simulink model "pump_simulator"  (R2020b)
settings: Solver=ode23t  StartTime=0.0  StopTime=sim_time  FixedStep=6.0  MaxStep=6.0  RelTol=1e-3
values from neighbouring files (symbols this model uses):
  bolus_size = 10    [insulin_pump.m]
  bolus_time = 3600*3    (= 10800)    [insulin_pump.m]
  damper_d1 = 5.0e4    (= 50000)    [insulin_pump.m]
  damper_d2 = 5    [insulin_pump.m]
  iis_area = pi*iis_diameter^2    (= 3.14159265359)    [insulin_pump.m]
  iis_elevation = 0    [insulin_pump.m]
  m_pulse_period = 3600 / n_pulses_per_hour    (= 180)    [insulin_pump.m]
  m_rotor_inertia = 0.051    [insulin_pump.m]
  m_volt = m_volt_nom    (= 3)    [insulin_pump.m]
  occ_area = iis_area    (= 3.14159265359)    [insulin_pump.m]
  occ_sw = 1    [insulin_pump.m]
  occ_tau = 2000    [insulin_pump.m]
  occ_time = s_locs(occ_idx)    [detect_occlusion.m]    (also in insulin_pump.m = 7200)
  piston_area = pi*reservoir_radius^2    [insulin_pump.m]
  piston_displacement_per_unit = U_per_ml / (piston_area)    [insulin_pump.m]
  piston_length = reservoir_len    (= 2.5)    [insulin_pump.m]
  pump_stop_time = 3600*6    (= 21600)    [insulin_pump.m]
  s_per_U = 60/flow_ml_min / 100    (= 12)    [insulin_pump.m]
  sim_time = 3600 * 10    (= 36000)    [insulin_pump.m]
  u_per_basal_pulse = basal_rate / n_pulses_per_hour    (= 0.05)    [insulin_pump.m]
libraries: fl_lib x38, nesl_utility x28, sh_lib x11, ee_lib x4, sdl_lib x3, simulink x1
(part 1 of 2)
Description:
  | Simulation of the physical mechanisms of an insulin pump.
settings Model: Creator=Mads  LastModifiedBy=Mads
settings DebuggingCC: AlgebraicLoopMsg=none

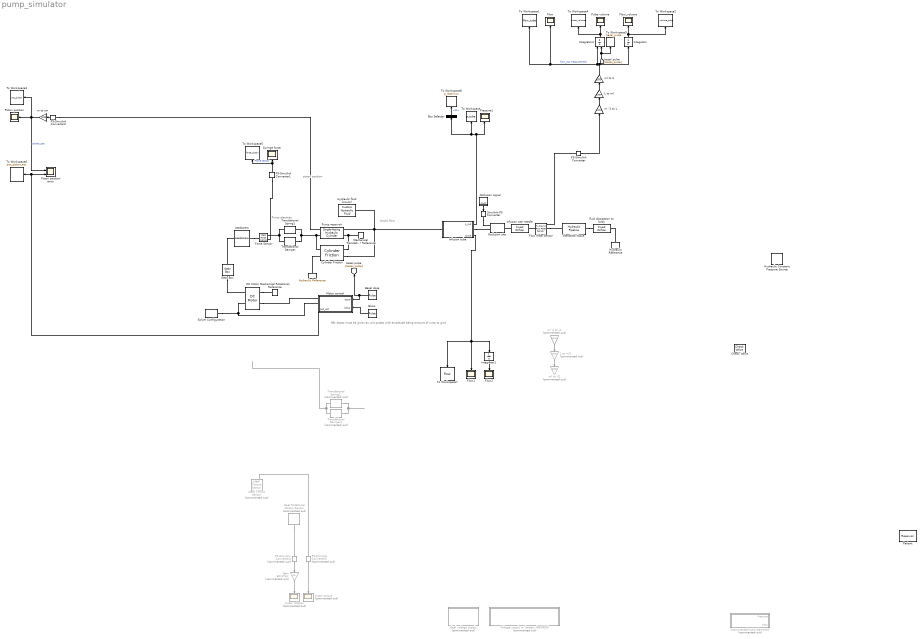
== system pump_simulator ==
  note: piston position
  note: NB: doses must be given as unit pulses with amplitude being amount of units to give
  note: Pump elasticity
  note: Insulin flow
  "  " : fl_lib/Hydraulic/Hydraulic Elements/Hydraulic Reference
  Basal dose : DiscretePulseGenerator  PulseType=Time based  Amplitude=u_per_basal_pulse  Period=m_pulse_period  PulseWidth=1e-11  PhaseDelay=10
  Bolus : DiscretePulseGenerator  PulseType=Time based  Amplitude=bolus_size  Period=sim_time  PulseWidth=1e-12  PhaseDelay=bolus_time
  Bus Selector : BusSelector  OutputSignals=p1
  Check Valve : sh_lib/Valves/Directional Valves/Check Valve  area_max=1e-4 m^2  pres_crack=0.3e5 Pa  pres_max=1.2e5 Pa  C_d=0.7  A_leak=1e-12 m^2  lam_spec=1  B_lam=0.999  Re_cr=12  dynamic=0  tau=0.1 s  area_init=1e-12 m^2
      settings: SourceProductBaseCode=SH  InternalSimscapePortConfiguration="{\"Bottom\":[],\"Left\":[{\"id\":\"A\",\"label\":\"A\",\"type\":\"foundation.hydraulic.hydraulic\"}],\"Right\":[{\"id\":\"B\",\"label\":\"B\",\"type\":\"foundation.hydraulic.hydraulic\"}],\"Top\":[]}"
  "Cylinder Friction " : sh_lib/Hydraulic Cylinders/Cylinder Friction  frc_preload=f_c N  fr_coef=f_cp N/Pa  frc_brkwy_coef=f_brk_c  visc_coef=f_v N/(m/s)  trans_coef=10000 s/m  vel_thr=v_limit cm/s  flow_rate_A_specify=off  flow_rate_A_priority=None  flow_rate_A=0 m^3/s  flow_rate_A_nominal_specify=off  flow_rate_A_nominal_unit=m^3/s  flow_rate_A_nominal_value=1  flow_rate_B_specify=off  flow_rate_B_priority=None  flow_rate_B=0 m^3/s  flow_rate_B_nominal_specify=off  flow_rate_B_nominal_unit=m^3/s  flow_rate_B_nominal_value=1  friction_force_specify=off  friction_force_priority=None  friction_force=0 N  friction_force_nominal_specify=off  friction_force_nominal_unit=N  friction_force_nominal_value=1  rel_velocity_specify=off  rel_velocity_priority=None  rel_velocity=0 m/s  rel_velocity_nominal_specify=off  rel_velocity_nominal_unit=m/s  rel_velocity_nominal_value=1
      settings: SourceProductBaseCode=SH  InternalSimscapePortConfiguration="{\"Bottom\":[],\"Left\":[{\"id\":\"A\",\"label\":\"A\",\"type\":\"foundation.hydraulic.hydraulic\"},{\"id\":\"C\",\"label\":\"C\",\"type\":\"foundation.mechanical.translational.translational\"}],\"Right\":[{\"id\":\"B\",\"label\":\"B\",\"type\":\"foundation.hydraulic.hydraulic\"},{\"id\":\"R\",\"label\":\"R\",\"type\":\"foundation.mechanical.translational.translational\"}],\"Top\":[]}"
  "DC Motor " : ee_lib/Electromechanical/Brushed Motors/DC Motor  field_option=ee.enum.field_option.pm  Rf=100 Ohm  Lf=1 H  Laf=0.15 H  If0=0 A  parameterization=ee.enum.dcparam_option.circuit_param  Ra=m_arm_res Ohm  La=m_arm_inductance uH  emf_or_torque=ee.enum.emf_or_torque.kv  Kv=m_back_emf V/rpm  Ki=6.876e-4 N*m/A  T_stall=0.24e-3 N*m  w_max=19100 rpm  w_rated=15000 rpm  P_rated=0.08 W  V_rated=1.5 V  J=m_rotor_inertia g*cm^2  lam_param=ee.enum.lam_param.damping  lam=0 N*m/(rad/s)  i_noload=0 A  V_i_noload=1.5 V  speed0=0 rpm  enable_fault_armature=ee.enum.faults.faultEnable.no  rev_faulted=1 / 3  G_faulted_armature=1e-5 S  fault_trigger_armature=ee.enum.faults.faultTrigger.temporal  t_fault_armature=1 s  max_permissible_current_armature=inf A  t_fail_on_current_armature=1 s  enable_fault_field=ee.enum.faults.faultEnable.no  G_faulted_field=1e-5 S  fault_trigger_field=ee.enum.faults.faultTrigger.temporal  t_fault_field=1 s  max_permissible_current_field=inf A  t_fail_on_current_field=1 s  fault_action=ee.enum.faults.faultAction.none  alpha=3.93e-3 1/K  Tmeas=25 degC  thermal_mass=100 J/K  initial_temperature=25 degC
  Flow : Scope
  Flow Rate Sensor : fl_lib/Hydraulic/Hydraulic Sensors/Hydraulic Flow Rate Sensor
  Flow1 : Scope
  Flow2 : Scope
  Flow_volume : Scope
  Force Sensor : fl_lib/Mechanical/Mechanical Sensors/Ideal Force Sensor
  Gain : Gain  Commented=on  Gain=60/(2*pi)
  "Gear Box " : fl_lib/Mechanical/Mechanisms/Gear Box  ratio=gear_ratio  t_in_specify=off  t_in_priority=None  t_in=0 N*m  t_in_nominal_specify=off  t_in_nominal_unit=N*m  t_in_nominal_value=1  t_out_specify=off  t_out_priority=None  t_out=0 N*m  t_out_nominal_specify=off  t_out_nominal_unit=N*m  t_out_nominal_value=1
  Hydraulic Constant Pressure Source : fl_lib/Hydraulic/Hydraulic Sources/Hydraulic Constant Pressure Source  commanded_pressure=patient_pressure Pa
      settings: SourceProductBaseCode=SS  InternalSimscapePortConfiguration="{\"Bottom\":[],\"Left\":[{\"id\":\"P\",\"label\":\"P\",\"type\":\"foundation.hydraulic.hydraulic\"}],\"Right\":[{\"id\":\"T\",\"label\":\"T\",\"type\":\"foundation.hydraulic.hydraulic\"}],\"Top\":[]}"
  "Hydraulic Reference " : fl_lib/Hydraulic/Hydraulic Elements/Hydraulic Reference
  Hydraulic fluid (insulin) : fl_lib/Hydraulic/Hydraulic Utilities/Custom Hydraulic Fluid  density=f_density kg/m^3  viscosity_kin=f_viscosity m^2/s  bulk=f_bmodulus GPa  alpha=0.005  range_error=2
      settings: SourceProductBaseCode=SS  InternalSimscapePortConfiguration="{\"Bottom\":[],\"Left\":[],\"Right\":[{\"id\":\"G\",\"label\":\"\",\"type\":\"foundation.hydraulic.hydraulic\"}],\"Top\":[]}"
  Ideal Rotational Motion Sensor : fl_lib/Mechanical/Mechanical Sensors/Ideal Rotational Motion Sensor  Commented=on  wrap_angle=simscape.enum.onoff.off  offset=0 rad
  Ideal Torque Sensor : fl_lib/Mechanical/Mechanical Sensors/Ideal Torque Sensor  Commented=on
  Ideal voltage supply : Subsystem  Commented=on
  Infusion site needle : sh_lib/Orifices/Fixed Orifice  area=cannula_area mm^2  C_d=0.7  lam_spec=1  B_lam=0.999  Re_cr=12  q_specify=off  q_priority=None  q=0.001 m^3/s  q_nominal_specify=off  q_nominal_unit=m^3/s  q_nominal_value=1  p_specify=on  p_priority=None  p=patient_pressure Pa  p_nominal_specify=off  p_nominal_unit=Pa  p_nominal_value=1
      settings: SourceProductBaseCode=SH  InternalSimscapePortConfiguration="{\"Bottom\":[],\"Left\":[{\"id\":\"A\",\"label\":\"A\",\"type\":\"foundation.hydraulic.hydraulic\"}],\"Right\":[{\"id\":\"B\",\"label\":\"B\",\"type\":\"foundation.hydraulic.hydraulic\"}],\"Top\":[]}"
  Infusion tube : Subsystem
      settings: PortSchema="{\"entries\":[{\"content\":{\"sides\":[{\"content\":{\"connectorIds\":[\"LConn1\"]},\"type\":\"ConnectorPlacement.EquallySpacedRectSide\",\"uuid\":\"e70f1e6d-11cd-47d8-af3d-56e3f4a89399\"},{\"content\":{\"connectorIds\":[\"Out1\",\"RConn1\",\"Out2\"],\"side\":\"RIGHT\"},\"type\":\"ConnectorPlacement.EquallySpacedRectSide\",\"uuid\":\"9455abbe-f67f-4bf6-bddd-a052e413b073\"},{\"content\":{\"connectorIds\":[],\"side\":\"TOP\"},\"type\":\"ConnectorPlacement.EquallySpacedRectSide\",\"uuid\":\"7aa9b125-01ea-4305-b1e3-58feaaf15538\"},{\"content\":{\"connectorIds\":[],\"side\":\"HIDDEN\"},\"type\":\"ConnectorPlacement.EquallySpacedRectSide\",\"uuid\":\"f40c7cd6-f259-44f6-9988-6f35709dc079\"}]},\"type\":\"ConnectorPlacement.EquallySpacedConnector\",\"uuid\":\"14f398f0-e936-4cfd-8d2f-f38c63dcd4d0\"}],\"packageUris\":[\"http://schema.mathworks.com/mf0/Connector/R2020b\"],\"version\":\"1.0\"}"
  Instrumented tube element3 : Subsystem  Commented=on
      settings: PortSchema="{\"entries\":[{\"content\":{\"sides\":[{\"content\":{\"connectorIds\":[\"LConn1\"]},\"type\":\"ConnectorPlacement.EquallySpacedRectSide\",\"uuid\":\"90113306-d748-46db-abc8-91bd69636f02\"},{\"content\":{\"connectorIds\":[\"Out1\",\"RConn1\",\"Out2\"],\"side\":\"RIGHT\"},\"type\":\"ConnectorPlacement.EquallySpacedRectSide\",\"uuid\":\"530dcab3-c363-40af-a674-d98a45a6a67f\"},{\"content\":{\"connectorIds\":[],\"side\":\"TOP\"},\"type\":\"ConnectorPlacement.EquallySpacedRectSide\",\"uuid\":\"49317322-7354-4795-83a8-239f759f7c98\"},{\"content\":{\"connectorIds\":[],\"side\":\"HIDDEN\"},\"type\":\"ConnectorPlacement.EquallySpacedRectSide\",\"uuid\":\"2a1d342c-23bd-4634-892a-7801d88aaf7b\"}]},\"type\":\"ConnectorPlacement.EquallySpacedConnector\",\"uuid\":\"7465f97d-dcd1-4a1e-863d-c659d9c7a8a5\"}],\"packageUris\":[\"http://schema.mathworks.com/mf0/Connector/R2020b\"],\"version\":\"1.0\"}"
  Integrator : Integrator
  Integrator1 : Integrator
  Integrator4 : Integrator  ExternalReset=rising
  Interstitial tissue : sh_lib/Pipelines/Hydraulic Pipeline  cs_type=1  d_in=pat_area m  area=1e-4 m^2  D_h=1.12e-2 m  s_factor=64  length=pat_len m  length_ad=pat_len m  roughness=15e-3 m  Re_lam=2000  Re_turb=4000  wall_type=2  pr_r_coef=pat_pressure_diameter m/Pa  time_const=pat_tau s  k_sh=1.4  initial_pressure=patient_pressure Pa
      settings: SourceProductBaseCode=SH  InternalSimscapePortConfiguration="{\"Bottom\":[],\"Left\":[{\"id\":\"A\",\"label\":\"A\",\"type\":\"foundation.hydraulic.hydraulic\"}],\"Right\":[{\"id\":\"B\",\"label\":\"B\",\"type\":\"foundation.hydraulic.hydraulic\"}],\"Top\":[]}"
  L to ml : Gain  Gain=1000
  L to ml1 : Gain  Commented=on  Gain=1000
  "Leadscrew " : sdl_lib/Gears/Rotational- Translational/Leadscrew  Lead=screw_lead cm  helix_type=sdl.enum.handedness.right  mu_visc=0 N*m/(rad/s)  friction_model=sdl.enum.gear_friction.constant  friction_parameterization=sdl.enum.frictionParameterization.geometry  lambda=15 deg  alpha=14.5 deg  fr_coeff=0.08  eff_sn=0.75  eff_ns=0.45  temperature_TLU=[280, 300, 320] K  efficiency_sn_TLU=[.75, .65, .6]  efficiency_ns_TLU=[.5, .45, .4]  pwr_thr=0.001 W  thermal_mass=50 J/K  temperature_specify=off  temperature_priority=High  temperature=300 K  temperature_nominal_specify=off  temperature_nominal_unit=K  temperature_nominal_value=1
      settings: SourceProductBaseCode=LD  InternalSimscapePortConfiguration="{\"Bottom\":[],\"Left\":[{\"id\":\"S\",\"label\":\"S\",\"type\":\"foundation.mechanical.rotational.rotational\"}],\"Right\":[{\"id\":\"N\",\"label\":\"N\",\"type\":\"foundation.mechanical.translational.translational\"}],\"Top\":[]}"
  Mechanical Rotational Reference : fl_lib/Mechanical/Rotational Elements/Mechanical Rotational Reference
  Mechanical Translational Reference : fl_lib/Mechanical/Translational Elements/Mechanical Translational Reference
  Motor control : Subsystem
      settings: PortSchema="{\"entries\":[{\"content\":{\"sides\":[{\"content\":{\"connectorIds\":[\"In1\",\"In2\"]},\"type\":\"ConnectorPlacement.EquallySpacedRectSide\",\"uuid\":\"d31ed946-0000-42cb-ba35-acda5a1e69b3\"},{\"content\":{\"connectorIds\":[\"RConn1\",\"RConn2\",\"Out1\"],\"side\":\"RIGHT\"},\"type\":\"ConnectorPlacement.EquallySpacedRectSide\",\"uuid\":\"d7d1f491-0bec-4320-8848-206ef8953605\"},{\"content\":{\"connectorIds\":[],\"side\":\"TOP\"},\"type\":\"ConnectorPlacement.EquallySpacedRectSide\",\"uuid\":\"d987aef5-87ba-45f9-8852-506aa6bf395c\"},{\"content\":{\"connectorIds\":[],\"side\":\"BOTTOM\"},\"type\":\"ConnectorPlacement.EquallySpacedRectSide\",\"uuid\":\"97925f89-ba97-42d0-b299-b4741c535cef\"},{\"content\":{\"connectorIds\":[],\"side\":\"HIDDEN\"},\"type\":\"ConnectorPlacement.EquallySpacedRectSide\",\"uuid\":\"d0973534-b90c-4eda-9531-680b99c38f66\"}]},\"type\":\"ConnectorPlacement.EquallySpacedConnector\",\"uuid\":\"4ca74101-9d3f-4e35-bde6-be4c600fefd9\"}],\"packageUris\":[\"http://schema.mathworks.com/mf0/Connector/R2020b\"],\"version\":\"1.0\"}"
  Occlusion signal : Subsystem
  Occlusion site : fl_lib/Hydraulic/Hydraulic Elements/Variable Area Hydraulic Orifice  C_d=0.7  min_area=1e-12 mm^2  lam_spec=1  B_lam=0.999  Re_cr=12  q_specify=off  q_priority=None  q=0.001 m^3/s  q_nominal_specify=off  q_nominal_unit=m^3/s  q_nominal_value=1  p_specify=off  p_priority=None  p=patient_pressure Pa  p_nominal_specify=off  p_nominal_unit=Pa  p_nominal_value=1
      settings: SourceProductBaseCode=SS  InternalSimscapePortConfiguration="{\"Bottom\":[],\"Left\":[{\"id\":\"AR\",\"label\":\"AR\",\"type\":\"input\"},{\"id\":\"A\",\"label\":\"A\",\"type\":\"foundation.hydraulic.hydraulic\"}],\"Right\":[{\"id\":\"B\",\"label\":\"B\",\"type\":\"foundation.hydraulic.hydraulic\"}],\"Top\":[]}"
  PS-Simulink Converter : nesl_utility/PS-Simulink Converter  PhysicalDomain=network_engine_domain  SubClassName=ps_output  LeftPortType=input  RightPortType=output  PseudoPeriodic=off  Frequencies=[]  Unit=inherit  AffineConversion=off
  PS-Simulink Converter1 : nesl_utility/PS-Simulink Converter  PhysicalDomain=network_engine_domain  SubClassName=ps_output  LeftPortType=input  RightPortType=output  PseudoPeriodic=off  Frequencies=[]  Unit=inherit  AffineConversion=off
  PS-Simulink Converter3 : nesl_utility/PS-Simulink Converter  PhysicalDomain=network_engine_domain  SubClassName=ps_output  LeftPortType=input  RightPortType=output  PseudoPeriodic=off  Frequencies=[]  Unit=inherit  AffineConversion=off
  PS-Simulink Converter4 : nesl_utility/PS-Simulink Converter  Commented=on  PhysicalDomain=network_engine_domain  SubClassName=ps_output  LeftPortType=input  RightPortType=output  PseudoPeriodic=off  Frequencies=[]  Unit=inherit  AffineConversion=off
  PS-Simulink Converter5 : nesl_utility/PS-Simulink Converter  Commented=on  PhysicalDomain=network_engine_domain  SubClassName=ps_output  LeftPortType=input  RightPortType=output  PseudoPeriodic=off  Frequencies=[]  Unit=inherit  AffineConversion=off
  Patient : sh_lib/Hydraulic Utilities/Reservoir  press=patient_pressure Pa  init_volume=5 l  ret_diam=cannula_area mm  loss_coeff=1
      settings: SourceProductBaseCode=SH  InternalSimscapePortConfiguration="{\"Bottom\":[],\"Left\":[{\"id\":\"V\",\"label\":\"V\",\"type\":\"output\"},{\"id\":\"P\",\"label\":\"P\",\"type\":\"foundation.hydraulic.hydraulic\"},{\"id\":\"R\",\"label\":\"R\",\"type\":\"foundation.hydraulic.hydraulic\"}],\"Right\":[],\"Top\":[]}"
  Piston position : Scope
  Piston position error : Scope  NumInputPorts=2
  Pressure1 : Scope
  Pulse volume : Scope
  Pump reservoir : sh_lib/Hydraulic Cylinders/Single-Acting Hydraulic Cylinder  area=piston_area cm^2  stroke=piston_length cm  init_pos=piston_length cm  dead_vol=piston_area*1e-12 cm^3  init_pressure=patient_pressure Pa  k_sh=1.4  stiff=1e6 N/m  D=150 N/(m/s)  hardstop_model=1  transition=4e-5 cm  or=2
      settings: SourceProductBaseCode=SH  InternalSimscapePortConfiguration="{\"Bottom\":[],\"Left\":[{\"id\":\"C\",\"label\":\"C\",\"type\":\"foundation.mechanical.translational.translational\"},{\"id\":\"A\",\"label\":\"A\",\"type\":\"foundation.hydraulic.hydraulic\"}],\"Right\":[{\"id\":\"R\",\"label\":\"R\",\"type\":\"foundation.mechanical.translational.translational\"},{\"id\":\"P\",\"label\":\"P\",\"type\":\"output\"}],\"Top\":[]}"
  Simulink-PS Converter : nesl_utility/Simulink-PS Converter  PhysicalDomain=network_engine_domain  SubClassName=ps_input  LeftPortType=input  RightPortType=output  PseudoPeriodic=off  Frequencies=[]  NoiseDistribution=none  NoiseParameters=[]  Unit=1  AffineConversion=off  FilteringAndDerivatives=provide  SimscapeFilterOrder=1  InputFilterTimeConstant=0.001  UdotUserProvided=0
  "Solver Configuration " : nesl_utility/Solver Configuration  PhysicalDomain=network_engine_domain  SubClassName=solver  LeftPortType=input  RightPortType=generic  Tones=[]  Harmonics=[]  SimulateNoise=off  Profile=off  UseLocalSampling=off  EnableSwitchedLinearOptims=on  FrequencyDomain=off  UseCCode=off  RelTol=0.001  AbsTol=1e-06  MinStep=1e-09  ToWorkspace=off  RevertToSquareIcSolve=off  NumHomotopyIterations=100  PhasorMode=off  PhasorModeNumHarmonics=1  DoDC=on  ResidualTolerance=1e-09  UseLocalSolver=off  LocalSolverChoice=NE_BACKWARD_EULER_ADVANCER  LocalSolverSampleTime=0.1  DoFixedCost=off  MaxNonlinIter=3  MaxModeIter=2  ComputeImpulses=off  ImpulseIterations=2  LinearAlgebra=auto  EquationFormulation=NE_TIME_EF  DelaysMemoryBudget=1024  AutomaticFiltering=on  FilteringTimeConstant=0.001  PartitionStorageMethod=AS_NEEDED  PartitionMemoryBudget=1024  PartitionMethod=ROBUST
  Syringe force : Scope
  To Workspace : ToWorkspace  VariableName=p_tube  SaveFormat=Timeseries  SampleTime=-1
  To Workspace1 : ToWorkspace  VariableName=flow_tube  SaveFormat=Timeseries  SampleTime=-1
  To Workspace2 : ToWorkspace  VariableName=volume_tube  SaveFormat=Timeseries  SampleTime=-1
  To Workspace3 : ToWorkspace  VariableName=pos_piston  SaveFormat=Timeseries  SampleTime=-1
  To Workspace4 : ToWorkspace  VariableName=pulse_volume  SaveFormat=Structure With Time  SampleTime=-1
  To Workspace5 : ToWorkspace  VariableName=force_piston  SaveFormat=Timeseries  SampleTime=-1
  To Workspace6 : ToWorkspace  VariableName=pos_piston_est  SaveFormat=Timeseries  SampleTime=-1
  To Workspace7 : ToWorkspace  VariableName=flow  SaveFormat=Timeseries  SampleTime=-1
  To Workspace8 : ToWorkspace  VariableName=p_reservoir  SaveFormat=Structure With Time  SampleTime=-1
  To Workspace9 : ToWorkspace  VariableName=basal_pulse  SaveFormat=Structure With Time  SampleTime=-1
  Translational Damper : sdl_lib/Couplings & Drives/Springs & Dampers/Translational Damper  D=damper_d1 N/(m/s)  enable_faults=0  b_fault=1e6 N/(m/s)  temporal_fault=0  fault_time=5 s  shock_fault=0  acceleration_limit=100 m/s^2  shock_limit=1  report_fault=1
      settings: SourceProductBaseCode=LD
  Translational Damper1 : sdl_lib/Couplings & Drives/Springs & Dampers/Translational Damper  Commented=on  D=damper_d2 N/(m/s)  enable_faults=0  b_fault=1e6 N/(m/s)  temporal_fault=0  fault_time=5 s  shock_fault=0  acceleration_limit=100 m/s^2  shock_limit=1  report_fault=1
      settings: SourceProductBaseCode=LD
  Translational Spring1 : fl_lib/Mechanical/Translational Elements/Translational Spring  spr_rate=spring_k1 N/m  v_specify=off  v_priority=None  v=0 m/s  v_nominal_specify=off  v_nominal_unit=m/s  v_nominal_value=1  f_specify=off  f_priority=None  f=0 N  f_nominal_specify=off  f_nominal_unit=N  f_nominal_value=1  x_specify=off  x_priority=High  x=1 mm  x_nominal_specify=off  x_nominal_unit=m  x_nominal_value=1
  Translational Spring2 : fl_lib/Mechanical/Translational Elements/Translational Spring  Commented=on  spr_rate=spring_k2 N/m  v_specify=off  v_priority=None  v=0 m/s  v_nominal_specify=off  v_nominal_unit=m/s  v_nominal_value=1  f_specify=off  f_priority=None  f=0 N  f_nominal_specify=off  f_nominal_unit=N  f_nominal_value=1  x_specify=off  x_priority=High  x=1 mm  x_nominal_specify=off  x_nominal_unit=m  x_nominal_value=1
  Voltage supply w/ battery (BROKEN) : Subsystem  Commented=on
  fluid dissipation to body : sh_lib/Orifices/Fixed Orifice  area=pat_dissipation mm^2  C_d=0.7  lam_spec=1  B_lam=0.999  Re_cr=12  q_specify=off  q_priority=None  q=0.001 m^3/s  q_nominal_specify=off  q_nominal_unit=m^3/s  q_nominal_value=1  p_specify=on  p_priority=None  p=patient_pressure Pa  p_nominal_specify=off  p_nominal_unit=Pa  p_nominal_value=1
      settings: SourceProductBaseCode=SH  InternalSimscapePortConfiguration="{\"Bottom\":[],\"Left\":[{\"id\":\"A\",\"label\":\"A\",\"type\":\"foundation.hydraulic.hydraulic\"}],\"Right\":[{\"id\":\"B\",\"label\":\"B\",\"type\":\"foundation.hydraulic.hydraulic\"}],\"Top\":[]}"
  m to cm : Gain  Gain=-100
  m^3 to L : Gain  Gain=1000
  m^3 to L1 : Gain  Commented=on  Gain=1000
  ml to U : Gain  Gain=100
  ml to U1 : Gain  Commented=on  Gain=100
  motor rotation : Scope  Commented=on
  motor torque : Scope  Commented=on
  wires:
  m to cm/1 -> Piston position error/1, To Workspace3/1, Piston position/1  "piston_pos"
  PS-Simulink Converter3/1 -> m to cm/1
  PS-Simulink Converter/1 -> m^3 to L/1
  m^3 to L/1 -> L to ml/1
  Integrator/1 -> To Workspace2/1, Flow_volume/1
  L to ml/1 -> ml to U/1
  ml to U/1 -> Flow/1, To Workspace1/1, Integrator4/1, Integrator/1  "flow_out measurement"
  Integrator1/1 -> Flow2/1
  Integrator4/1 -> To Workspace4/1, Pulse volume/1
  [basal_pulse] -> To Workspace9/1, Integrator4/2
  m^3 to L1/1 -> L to ml1/1
  L to ml1/1 -> ml to U1/1
  Occlusion signal/1(Out2) -> Simulink-PS Converter/1
  Bus Selector/1 -> To Workspace8/1  "<p1>"
  Gain/1 -> motor rotation/1
  PS-Simulink Converter5/1 -> motor torque/1
  PS-Simulink Converter4/1 -> Gain/1
  PS-Simulink Converter1/1 -> To Workspace5/1, Syringe force/1  "Force sensor"
  Bolus/1 -> Motor control/2(bolus)
  Infusion tube/1(p_out) -> Bus Selector/1, To Workspace/1, Pressure1/1
  Infusion tube/2(q_out) -> To Workspace7/1, Integrator1/1, Flow1/1
  Basal dose/1 -> [basal_pulse], Motor control/1(basal)
  Motor control/1(pos_est) -> To Workspace6/1, Piston position error/2
  connections:
  Infusion site needle/LConn1 -- Occlusion site/RConn1
  Simulink-PS Converter/RConn1 -- Occlusion site/LConn1
  Flow Rate Sensor/LConn1 -- Infusion site needle/RConn1
  Interstitial tissue/RConn1 -- fluid dissipation to body/LConn1
  "Hydraulic Reference "/LConn1 -- fluid dissipation to body/RConn1
  "DC Motor "/RConn2 -- Mechanical Rotational Reference/LConn1
  "Leadscrew "/RConn1 -- Force Sensor/LConn1
  "Cylinder Friction "/LConn2 -- Mechanical Translational Reference/LConn1 -- Pump reservoir/LConn1
  "  "/LConn1 -- "Cylinder Friction "/RConn1
  "Leadscrew "/LConn1 -- "Gear Box "/RConn1
  Force Sensor/RConn1 -- Translational Damper/LConn1 -- Translational Spring1/LConn1
  Translational Spring1/RConn1 -- Translational Damper/RConn1 -- "Cylinder Friction "/RConn2 -- Pump reservoir/RConn1
  "Cylinder Friction "/LConn1 -- Infusion tube/LConn1 -- Pump reservoir/LConn2 -- Hydraulic fluid (insulin)/RConn1
  Infusion tube/RConn1 -- Occlusion site/LConn2
  "Gear Box "/LConn1 -- "DC Motor "/LConn2
  Flow Rate Sensor/RConn2 -- Interstitial tissue/LConn1
  Ideal Rotational Motion Sensor/RConn2 -- PS-Simulink Converter4/LConn1
  PS-Simulink Converter5/LConn1 -- Ideal Torque Sensor/RConn2
  Translational Damper1/LConn1 -- Translational Spring2/LConn1
  Translational Damper1/RConn1 -- Translational Spring2/RConn1
  "DC Motor "/LConn1 -- "Solver Configuration "/RConn1 -- Motor control/RConn2
  "DC Motor "/RConn1 -- Motor control/RConn1
  PS-Simulink Converter/LConn1 -- Flow Rate Sensor/RConn1
  PS-Simulink Converter1/LConn1 -- Force Sensor/RConn2
  PS-Simulink Converter3/LConn1 -- Pump reservoir/RConn2

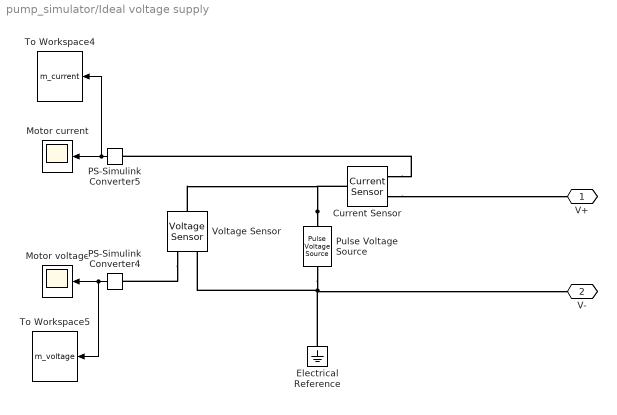
== system pump_simulator/Ideal voltage supply ==
  "Current Sensor " : fl_lib/Electrical/Electrical Sensors/Current Sensor
  "Electrical Reference " : fl_lib/Electrical/Electrical Elements/Electrical Reference
  Motor current : Scope
  Motor voltage : Scope
  PS-Simulink Converter4 : nesl_utility/PS-Simulink Converter  PhysicalDomain=network_engine_domain  SubClassName=ps_output  LeftPortType=input  RightPortType=output  PseudoPeriodic=off  Frequencies=[]  Unit=inherit  AffineConversion=off
  PS-Simulink Converter5 : nesl_utility/PS-Simulink Converter  PhysicalDomain=network_engine_domain  SubClassName=ps_output  LeftPortType=input  RightPortType=output  PseudoPeriodic=off  Frequencies=[]  Unit=inherit  AffineConversion=off
  "Pulse Voltage Source " : ee_lib/Additional Components/SPICE Sources/Pulse Voltage Source  V1=0 V  V2=m_volt V  TD=m_pulse_width s  TR=1e-9 s  TF=1e-9 s  PW=m_pulse_width s  PER=m_pulse_period s
      settings: SourceProductBaseCode=PS  InternalSimscapePortConfiguration="{\"Bottom\":[],\"Left\":[{\"id\":\"p\",\"label\":\"\",\"type\":\"foundation.electrical.electrical\"}],\"Right\":[{\"id\":\"n\",\"label\":\"\",\"type\":\"foundation.electrical.electrical\"}],\"Top\":[]}"
  To Workspace4 : ToWorkspace  VariableName=m_current  SaveFormat=Timeseries  SampleTime=-1
  To Workspace5 : ToWorkspace  VariableName=m_voltage  SaveFormat=Timeseries  SampleTime=-1
  "Voltage Sensor " : fl_lib/Electrical/Electrical Sensors/Voltage Sensor
  V+ : PMIOPort  Side=Right
  V- : PMIOPort  Port=2  Side=Right
  wires:
  PS-Simulink Converter4/1 -> To Workspace5/1, Motor voltage/1
  PS-Simulink Converter5/1 -> To Workspace4/1, Motor current/1
  connections:
  "Voltage Sensor "/RConn1 -- PS-Simulink Converter4/LConn1
  "Pulse Voltage Source "/LConn1 -- "Voltage Sensor "/LConn1 -- "Current Sensor "/LConn1
  "Current Sensor "/RConn1 -- PS-Simulink Converter5/LConn1
  "Current Sensor "/RConn2 -- V+/RConn1
  "Pulse Voltage Source "/RConn1 -- "Electrical Reference "/LConn1 -- V-/RConn1 -- "Voltage Sensor "/RConn2

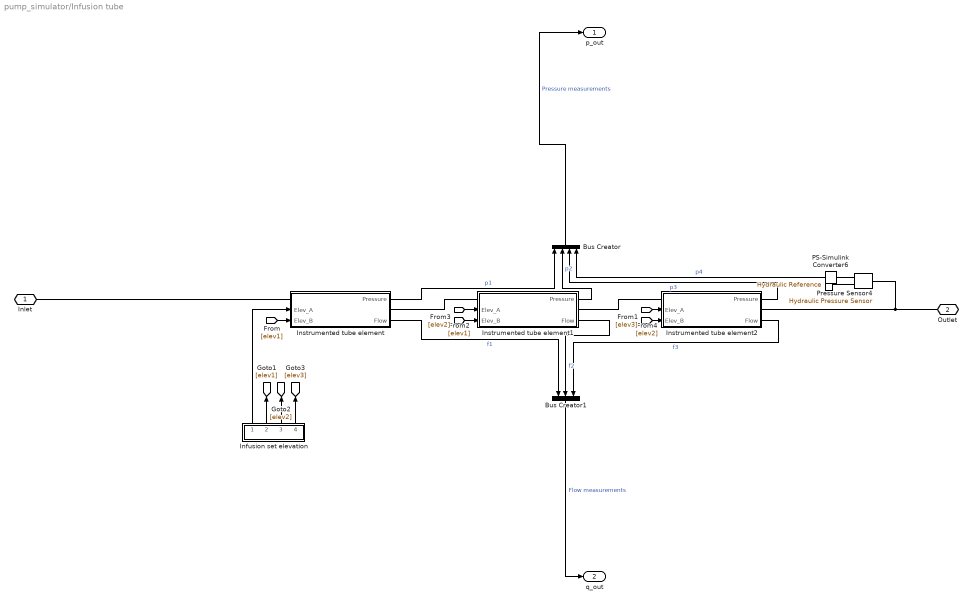
== system pump_simulator/Infusion tube ==
  " " : fl_lib/Hydraulic/Hydraulic Elements/Hydraulic Reference
  Bus Creator : BusCreator  Inputs=4
  Bus Creator1 : BusCreator  Inputs=3
  Infusion set elevation : Subsystem
  Instrumented tube element : Subsystem
      settings: PortSchema="{\"entries\":[{\"content\":{\"sides\":[{\"content\":{\"connectorIds\":[\"LConn1\",\"In1\",\"In2\"]},\"type\":\"ConnectorPlacement.EquallySpacedRectSide\",\"uuid\":\"90113306-d748-46db-abc8-91bd69636f02\"},{\"content\":{\"connectorIds\":[\"Out1\",\"RConn1\",\"Out2\"],\"side\":\"RIGHT\"},\"type\":\"ConnectorPlacement.EquallySpacedRectSide\",\"uuid\":\"530dcab3-c363-40af-a674-d98a45a6a67f\"},{\"content\":{\"connectorIds\":[],\"side\":\"TOP\"},\"type\":\"ConnectorPlacement.EquallySpacedRectSide\",\"uuid\":\"49317322-7354-4795-83a8-239f759f7c98\"},{\"content\":{\"connectorIds\":[],\"side\":\"HIDDEN\"},\"type\":\"ConnectorPlacement.EquallySpacedRectSide\",\"uuid\":\"2a1d342c-23bd-4634-892a-7801d88aaf7b\"}]},\"type\":\"ConnectorPlacement.EquallySpacedConnector\",\"uuid\":\"7465f97d-dcd1-4a1e-863d-c659d9c7a8a5\"}],\"packageUris\":[\"http://schema.mathworks.com/mf0/Connector/R2020b\"],\"version\":\"1.0\"}"
  Instrumented tube element1 : Subsystem
      settings: PortSchema="{\"entries\":[{\"content\":{\"sides\":[{\"content\":{\"connectorIds\":[\"LConn1\",\"In1\",\"In2\"]},\"type\":\"ConnectorPlacement.EquallySpacedRectSide\",\"uuid\":\"90113306-d748-46db-abc8-91bd69636f02\"},{\"content\":{\"connectorIds\":[\"Out1\",\"RConn1\",\"Out2\"],\"side\":\"RIGHT\"},\"type\":\"ConnectorPlacement.EquallySpacedRectSide\",\"uuid\":\"530dcab3-c363-40af-a674-d98a45a6a67f\"},{\"content\":{\"connectorIds\":[],\"side\":\"TOP\"},\"type\":\"ConnectorPlacement.EquallySpacedRectSide\",\"uuid\":\"49317322-7354-4795-83a8-239f759f7c98\"},{\"content\":{\"connectorIds\":[],\"side\":\"HIDDEN\"},\"type\":\"ConnectorPlacement.EquallySpacedRectSide\",\"uuid\":\"2a1d342c-23bd-4634-892a-7801d88aaf7b\"}]},\"type\":\"ConnectorPlacement.EquallySpacedConnector\",\"uuid\":\"7465f97d-dcd1-4a1e-863d-c659d9c7a8a5\"}],\"packageUris\":[\"http://schema.mathworks.com/mf0/Connector/R2020b\"],\"version\":\"1.0\"}"
  Instrumented tube element2 : Subsystem
      settings: PortSchema="{\"entries\":[{\"content\":{\"sides\":[{\"content\":{\"connectorIds\":[\"LConn1\",\"In1\",\"In2\"]},\"type\":\"ConnectorPlacement.EquallySpacedRectSide\",\"uuid\":\"90113306-d748-46db-abc8-91bd69636f02\"},{\"content\":{\"connectorIds\":[\"Out1\",\"RConn1\",\"Out2\"],\"side\":\"RIGHT\"},\"type\":\"ConnectorPlacement.EquallySpacedRectSide\",\"uuid\":\"530dcab3-c363-40af-a674-d98a45a6a67f\"},{\"content\":{\"connectorIds\":[],\"side\":\"TOP\"},\"type\":\"ConnectorPlacement.EquallySpacedRectSide\",\"uuid\":\"49317322-7354-4795-83a8-239f759f7c98\"},{\"content\":{\"connectorIds\":[],\"side\":\"HIDDEN\"},\"type\":\"ConnectorPlacement.EquallySpacedRectSide\",\"uuid\":\"2a1d342c-23bd-4634-892a-7801d88aaf7b\"}]},\"type\":\"ConnectorPlacement.EquallySpacedConnector\",\"uuid\":\"7465f97d-dcd1-4a1e-863d-c659d9c7a8a5\"}],\"packageUris\":[\"http://schema.mathworks.com/mf0/Connector/R2020b\"],\"version\":\"1.0\"}"
  PS-Simulink Converter6 : nesl_utility/PS-Simulink Converter  PhysicalDomain=network_engine_domain  SubClassName=ps_output  LeftPortType=input  RightPortType=output  PseudoPeriodic=off  Frequencies=[]  Unit=inherit  AffineConversion=off
  Pressure Sensor4 : fl_lib/Hydraulic/Hydraulic Sensors/Hydraulic Pressure Sensor
  Inlet : PMIOPort  Side=Left
  Outlet : PMIOPort  Port=2  Side=Right
  p_out : Outport
  q_out : Outport  Port=2
  wires:
  Infusion set elevation/2(elev1) -> [elev1]
  Instrumented tube element1/1(Pressure) -> Bus Creator/2  "p2"
  Instrumented tube element2/2(Flow) -> Bus Creator1/3  "f3"
  [elev1] -> Instrumented tube element1/1(Elev_A)
  Instrumented tube element2/1(Pressure) -> Bus Creator/3  "p3"
  Instrumented tube element/1(Pressure) -> Bus Creator/1  "p1"
  [elev2] -> Instrumented tube element2/1(Elev_A)
  Infusion set elevation/1(elev0) -> Instrumented tube element/1(Elev_A)
  Infusion set elevation/3(elev2) -> [elev2]
  [elev1] -> Instrumented tube element/2(Elev_B)
  Infusion set elevation/4(elev_ref) -> [elev3]
  PS-Simulink Converter6/1 -> Bus Creator/4  "p4"
  [elev2] -> Instrumented tube element1/2(Elev_B)
  Instrumented tube element/2(Flow) -> Bus Creator1/1  "f1"
  Instrumented tube element1/2(Flow) -> Bus Creator1/2  "f2"
  [elev3] -> Instrumented tube element2/2(Elev_B)
  Bus Creator/1 -> p_out/1  "Pressure measurements"
  Bus Creator1/1 -> q_out/1  "Flow measurements"
  connections:
  Instrumented tube element/RConn1 -- Instrumented tube element1/LConn1
  Instrumented tube element1/RConn1 -- Instrumented tube element2/LConn1
  Pressure Sensor4/RConn1 -- " "/LConn1
  Pressure Sensor4/LConn1 -- Outlet/RConn1 -- Instrumented tube element2/RConn1
  PS-Simulink Converter6/LConn1 -- Pressure Sensor4/RConn2
  Inlet/RConn1 -- Instrumented tube element/LConn1

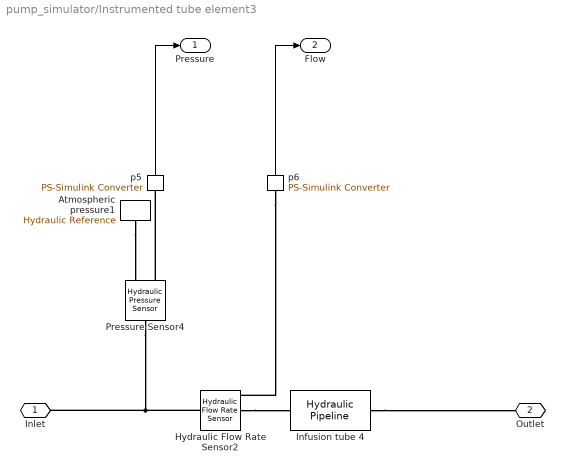
== system pump_simulator/Instrumented tube element3 ==
  Atmospheric pressure1 : fl_lib/Hydraulic/Hydraulic Elements/Hydraulic Reference
  Hydraulic Flow Rate Sensor2 : fl_lib/Hydraulic/Hydraulic Sensors/Hydraulic Flow Rate Sensor
  Infusion tube 4 : sh_lib/Pipelines/Hydraulic Pipeline  cs_type=1  d_in=iis_diameter mm  area=1e-4 m^2  D_h=1.12e-2 m  s_factor=64  length=iis_element_len cm  length_ad=1 m  roughness=15e-6 m  Re_lam=2000  Re_turb=4000  wall_type=2  pr_r_coef=iis_pres_dia_value m/Pa  time_const=0.01 s  k_sh=1.4  initial_pressure=patient_pressure Pa
      settings: SourceProductBaseCode=SH  InternalSimscapePortConfiguration="{\"Bottom\":[],\"Left\":[{\"id\":\"A\",\"label\":\"A\",\"type\":\"foundation.hydraulic.hydraulic\"}],\"Right\":[{\"id\":\"B\",\"label\":\"B\",\"type\":\"foundation.hydraulic.hydraulic\"}],\"Top\":[]}"
  Pressure Sensor4 : fl_lib/Hydraulic/Hydraulic Sensors/Hydraulic Pressure Sensor
  p5 : nesl_utility/PS-Simulink Converter  PhysicalDomain=network_engine_domain  SubClassName=ps_output  LeftPortType=input  RightPortType=output  PseudoPeriodic=off  Frequencies=[]  Unit=inherit  AffineConversion=off
  p6 : nesl_utility/PS-Simulink Converter  PhysicalDomain=network_engine_domain  SubClassName=ps_output  LeftPortType=input  RightPortType=output  PseudoPeriodic=off  Frequencies=[]  Unit=inherit  AffineConversion=off
  Inlet : PMIOPort  Side=Left
  Outlet : PMIOPort  Port=2  Side=Right
  Pressure : Outport
  Flow : Outport  Port=2
  wires:
  p6/1 -> Flow/1
  p5/1 -> Pressure/1
  connections:
  Hydraulic Flow Rate Sensor2/LConn1 -- Pressure Sensor4/LConn1 -- Inlet/RConn1
  p6/LConn1 -- Hydraulic Flow Rate Sensor2/RConn1
  Infusion tube 4/RConn1 -- Outlet/RConn1
  Atmospheric pressure1/LConn1 -- Pressure Sensor4/RConn1
  Hydraulic Flow Rate Sensor2/RConn2 -- Infusion tube 4/LConn1
  Pressure Sensor4/RConn2 -- p5/LConn1

== system pump_simulator/Motor control ==
  basal : Inport
  bolus : Inport  Port=2
  Motor control : Subsystem
  Power supply : Subsystem
  V- : PMIOPort  Side=Right
  V+ : PMIOPort  Port=2  Side=Right
  pos_est : Outport
  wires:
  Motor control/2(v_ref) -> Power supply/1(V_ref)
  basal/1 -> Motor control/1(Basal dose)
  bolus/1 -> Motor control/2(Bolus)
  Motor control/1(piston_pos_est) -> pos_est/1  "piston_pos_est"
  connections:
  V+/RConn1 -- Power supply/RConn1
  V-/RConn1 -- Power supply/RConn2

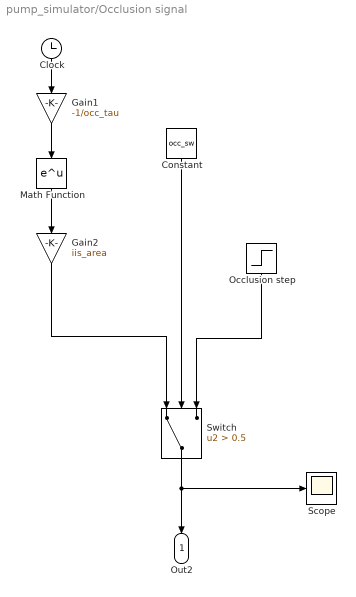
== system pump_simulator/Occlusion signal ==
  Clock : Clock
  Constant : Constant  Value=occ_sw
  Gain1 : Gain  Gain=-1/occ_tau
  Gain2 : Gain  Gain=iis_area
  Math Function : Math  SaturateOnIntegerOverflow=on
  Occlusion step : Step  Time=occ_time  Before=iis_area  After=occ_area  SampleTime=0
  Scope : Scope
  Switch : Switch  Criteria=u2 > Threshold  Threshold=0.5
  Out2 : Outport
  wires:
  Gain1/1 -> Math Function/1
  Clock/1 -> Gain1/1
  Math Function/1 -> Gain2/1
  Gain2/1 -> Switch/1
  Occlusion step/1 -> Switch/3
  Switch/1 -> Scope/1, Out2/1
  Constant/1 -> Switch/2

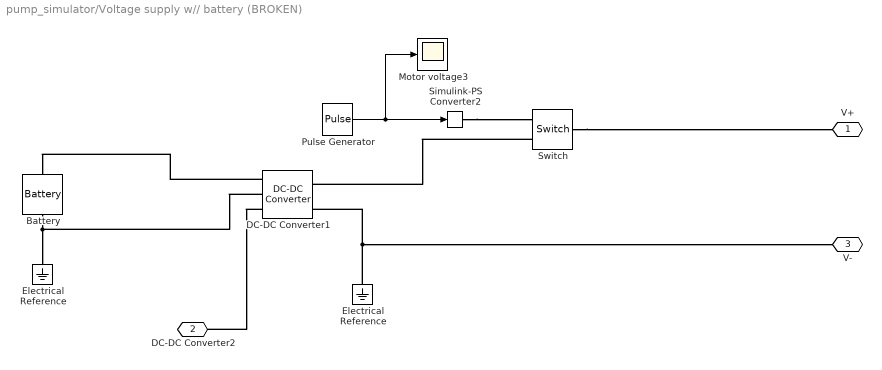
== system pump_simulator/Voltage supply w// battery (BROKEN) ==
  Battery : ee_lib/Sources/Battery  Vnom=3 V  prm_dir=1  R1_dis=2 Ohm  R1_ch=2 Ohm  R1=2 Ohm  prm_AH=1  AH=50 hr*A  V1=11.5 V  AH1=25 hr*A  prm_R2=1  R2=2000 Ohm  prm_dyn=1  Rp1=0.005 Ohm  tau1=30 s  Rp2=0.005 Ohm  tau2=30 s  Rp3=0.005 Ohm  tau3=30 s  Rp4=0.005 Ohm  tau4=30 s  Rp5=0.005 Ohm  tau5=30 s  prm_fade=1  N_fade=100  AH_fade=45 hr*A  R1_fade=2.02 Ohm  R1_ch_fade=2.02 Ohm  V1_fade=10.35 V  i_specify=off  i_priority=None  i=0 A  i_nominal_specify=off  i_nominal_unit=A  i_nominal_value=1  v_specify=off  v_priority=None  v=0 V  v_nominal_specify=off  v_nominal_unit=V  v_nominal_value=1  charge_specify=off  charge_priority=High  charge=50 hr*A  charge_nominal_specify=off  charge_nominal_unit=hr*A  charge_nominal_value=1  num_cycles_specify=off  num_cycles_priority=High  num_cycles=0  num_cycles_nominal_specify=off  num_cycles_nominal_unit=1  num_cycles_nominal_value=1  thermal_mass=30000 J/K  Tmeas=298.15 K  Vnom_T2=12 V  R1_T2=2.2 Ohm  R1_T2_dis=2.2 Ohm  R1_T2_ch=2.2 Ohm  V1_T2=11.4 V  R2_T2=2200 Ohm  Rp1_T2=0.005 Ohm  tau1_T2=30 s  Rp2_T2=0.005 Ohm  tau2_T2=30 s  Rp3_T2=0.005 Ohm  tau3_T2=30 s  Rp4_T2=0.005 Ohm  tau4_T2=30 s  Rp5_T2=0.005 Ohm  tau5_T2=30 s  Tmeas2=273.15 K  temperature_specify=off  temperature_priority=High  temperature=298.15 K  temperature_nominal_specify=off  temperature_nominal_unit=K  temperature_nominal_value=1
  DC-DC Converter1 : ee_lib/Semiconductors & Converters/Converters/DC-DC Converter  Vref_option=ee.enum.converters.voltageref.internal  v_ref=6 V  P_rated=10 W  droop_param=1  droop=0.1 V/A  droop_percent=2  reversible=0  efficiency=80  P_fixed=1 W  model_dynamics=0  tau=0.02 s  v_ini=10 V  G_diode=1e-8 1/Ohm  i1_max=2 A  fault_condition=1  fault_threshold=0.5  thermal_mass=100 J/K  initial_temperature=298.15 K
      settings: SourceProductBaseCode=PS  InternalSimscapePortConfiguration="{\"Bottom\":[],\"Left\":[{\"id\":\"p1\",\"label\":\"1+\",\"type\":\"foundation.electrical.electrical\"},{\"id\":\"n1\",\"label\":\"1-\",\"type\":\"foundation.electrical.electrical\"},{\"id\":\"F\",\"label\":\"F\",\"type\":\"input\"}],\"Right\":[{\"id\":\"p2\",\"label\":\"2+\",\"type\":\"foundation.electrical.electrical\"},{\"id\":\"n2\",\"label\":\"2-\",\"type\":\"foundation.electrical.electrical\"}],\"Top\":[]}"
  Electrical Reference : fl_lib/Electrical/Electrical Elements/Electrical Reference
  "Electrical Reference " : fl_lib/Electrical/Electrical Elements/Electrical Reference
  Motor voltage3 : Scope
  Pulse Generator : DiscretePulseGenerator  PulseType=Time based  Period=10  PulseWidth=50  PhaseDelay=10
  Simulink-PS Converter2 : nesl_utility/Simulink-PS Converter  PhysicalDomain=network_engine_domain  SubClassName=ps_input  LeftPortType=input  RightPortType=output  PseudoPeriodic=off  Frequencies=[]  NoiseDistribution=none  NoiseParameters=[]  Unit=1  AffineConversion=off  FilteringAndDerivatives=provide  SimscapeFilterOrder=1  InputFilterTimeConstant=0.001  UdotUserProvided=0
  Switch : fl_lib/Electrical/Electrical Elements/Switch  R_closed=0.01 Ohm  G_open=1e-8 1/Ohm  Threshold=0.5  i_specify=off  i_priority=None  i=0 A  i_nominal_specify=off  i_nominal_unit=A  i_nominal_value=1  v_specify=off  v_priority=None  v=0 V  v_nominal_specify=off  v_nominal_unit=V  v_nominal_value=1
  V+ : PMIOPort  Side=Right
  DC-DC Converter2 : PMIOPort  Port=2  Side=Left
  V- : PMIOPort  Port=3  Side=Right
  wires:
  Pulse Generator/1 -> Motor voltage3/1, Simulink-PS Converter2/1
  connections:
  Simulink-PS Converter2/RConn1 -- Switch/RConn1
  DC-DC Converter1/LConn3 -- DC-DC Converter2/RConn1
  DC-DC Converter1/LConn1 -- Battery/LConn1
  Electrical Reference/LConn1 -- DC-DC Converter1/RConn2 -- V-/RConn1
  Switch/RConn2 -- DC-DC Converter1/RConn1
  Battery/RConn1 -- "Electrical Reference "/LConn1 -- DC-DC Converter1/LConn2
  Switch/LConn1 -- V+/RConn1

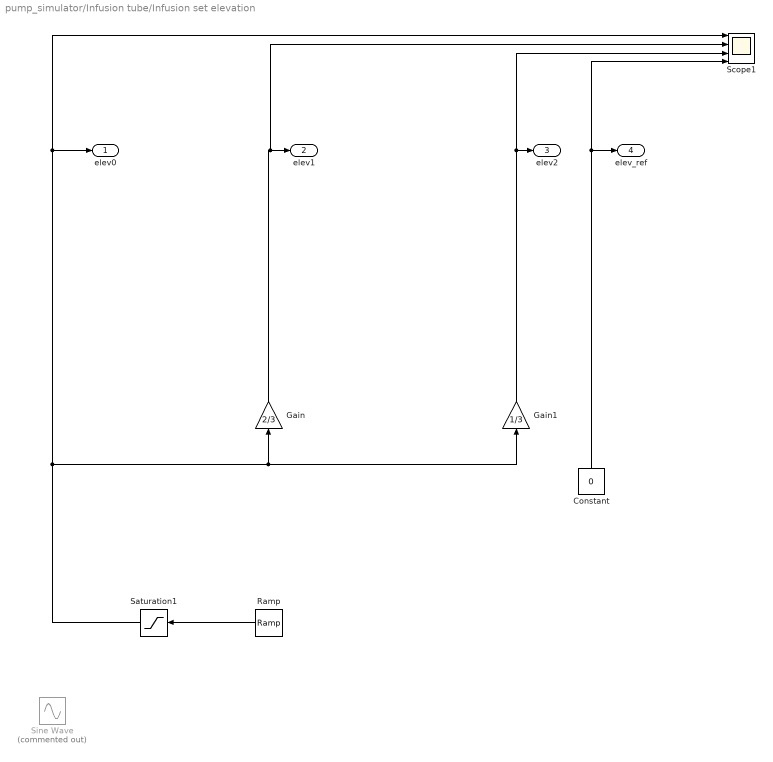
== system pump_simulator/Infusion tube/Infusion set elevation ==
  Constant : Constant  Value=0
  Gain : Gain  Gain=2/3
  Gain1 : Gain  Gain=1/3
  Ramp : simulink/Sources/Ramp  slope=0.25 * sign(iis_elevation)  start=5  InitialOutput=0
  Saturation1 : Saturate  UpperLimit=abs(iis_elevation)  LowerLimit=-abs(iis_elevation)
  Scope1 : Scope  NumInputPorts=4
  Sine Wave : Sin  Commented=on  Amplitude=iis_elevation  Frequency=0.01  SampleTime=0
  elev0 : Outport
  elev1 : Outport  Port=2
  elev2 : Outport  Port=3
  elev_ref : Outport  Port=4
  wires:
  Ramp/1 -> Saturation1/1
  Gain1/1 -> Scope1/3, elev2/1
  Constant/1 -> Scope1/4, elev_ref/1
  Gain/1 -> Scope1/2, elev1/1
  Saturation1/1 -> Gain1/1, Gain/1, Scope1/1, elev0/1

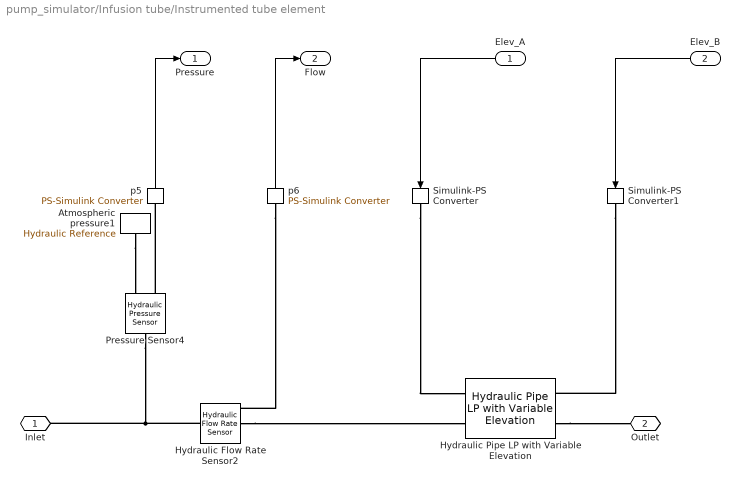
== system pump_simulator/Infusion tube/Instrumented tube element ==
  Elev_A : Inport
  Elev_B : Inport  Port=2
  Atmospheric pressure1 : fl_lib/Hydraulic/Hydraulic Elements/Hydraulic Reference
  Hydraulic Flow Rate Sensor2 : fl_lib/Hydraulic/Hydraulic Sensors/Hydraulic Flow Rate Sensor
  Hydraulic Pipe LP with Variable Elevation : sh_lib/Low-Pressure Blocks/Hydraulic Pipe LP with Variable Elevation  cs_type=1  d_in=iis_diameter mm  area=1e-4 m^2  D_h=1.12e-2 m  s_factor=64  length=iis_element_len m  length_ad=1 m  roughness=15e-6 m  Re_lam=2000  Re_turb=4000  g=9.80665 m/s^2  wall_type=2  pr_r_coef=iis_pres_dia_value m/Pa  time_const=0.01 s  k_sh=1.4  p0=patient_pressure Pa
      settings: SourceProductBaseCode=SH  InternalSimscapePortConfiguration="{\"Bottom\":[],\"Left\":[{\"id\":\"el_A\",\"label\":\"el_A\",\"type\":\"input\"},{\"id\":\"A\",\"label\":\"A\",\"type\":\"foundation.hydraulic.hydraulic\"}],\"Right\":[{\"id\":\"el_B\",\"label\":\"el_B\",\"type\":\"input\"},{\"id\":\"B\",\"label\":\"B\",\"type\":\"foundation.hydraulic.hydraulic\"}],\"Top\":[]}"
  Pressure Sensor4 : fl_lib/Hydraulic/Hydraulic Sensors/Hydraulic Pressure Sensor
  Simulink-PS Converter : nesl_utility/Simulink-PS Converter  PhysicalDomain=network_engine_domain  SubClassName=ps_input  LeftPortType=input  RightPortType=output  PseudoPeriodic=off  Frequencies=[]  NoiseDistribution=none  NoiseParameters=[]  Unit=1  AffineConversion=off  FilteringAndDerivatives=provide  SimscapeFilterOrder=1  InputFilterTimeConstant=0.001  UdotUserProvided=0
  Simulink-PS Converter1 : nesl_utility/Simulink-PS Converter  PhysicalDomain=network_engine_domain  SubClassName=ps_input  LeftPortType=input  RightPortType=output  PseudoPeriodic=off  Frequencies=[]  NoiseDistribution=none  NoiseParameters=[]  Unit=1  AffineConversion=off  FilteringAndDerivatives=provide  SimscapeFilterOrder=1  InputFilterTimeConstant=0.001  UdotUserProvided=0
  p5 : nesl_utility/PS-Simulink Converter  PhysicalDomain=network_engine_domain  SubClassName=ps_output  LeftPortType=input  RightPortType=output  PseudoPeriodic=off  Frequencies=[]  Unit=inherit  AffineConversion=off
  p6 : nesl_utility/PS-Simulink Converter  PhysicalDomain=network_engine_domain  SubClassName=ps_output  LeftPortType=input  RightPortType=output  PseudoPeriodic=off  Frequencies=[]  Unit=inherit  AffineConversion=off
  Inlet : PMIOPort  Side=Left
  Outlet : PMIOPort  Port=2  Side=Right
  Pressure : Outport
  Flow : Outport  Port=2
  wires:
  p6/1 -> Flow/1
  p5/1 -> Pressure/1
  Elev_A/1 -> Simulink-PS Converter/1
  Elev_B/1 -> Simulink-PS Converter1/1
  connections:
  Pressure Sensor4/LConn1 -- Inlet/RConn1 -- Hydraulic Flow Rate Sensor2/LConn1
  p6/LConn1 -- Hydraulic Flow Rate Sensor2/RConn1
  Atmospheric pressure1/LConn1 -- Pressure Sensor4/RConn1
  Pressure Sensor4/RConn2 -- p5/LConn1
  Hydraulic Pipe LP with Variable Elevation/RConn2 -- Outlet/RConn1
  Hydraulic Flow Rate Sensor2/RConn2 -- Hydraulic Pipe LP with Variable Elevation/LConn2
  Simulink-PS Converter/RConn1 -- Hydraulic Pipe LP with Variable Elevation/LConn1
  Simulink-PS Converter1/RConn1 -- Hydraulic Pipe LP with Variable Elevation/RConn1

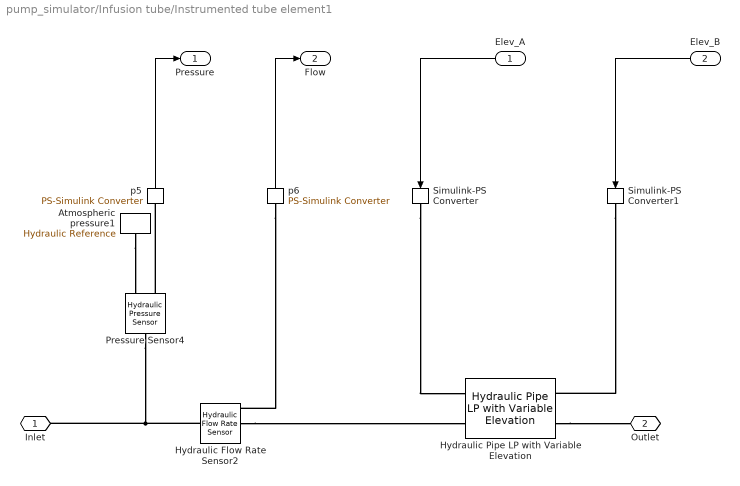
== system pump_simulator/Infusion tube/Instrumented tube element1 ==
  Elev_A : Inport
  Elev_B : Inport  Port=2
  Atmospheric pressure1 : fl_lib/Hydraulic/Hydraulic Elements/Hydraulic Reference
  Hydraulic Flow Rate Sensor2 : fl_lib/Hydraulic/Hydraulic Sensors/Hydraulic Flow Rate Sensor
  Hydraulic Pipe LP with Variable Elevation : sh_lib/Low-Pressure Blocks/Hydraulic Pipe LP with Variable Elevation  cs_type=1  d_in=iis_diameter mm  area=1e-4 m^2  D_h=1.12e-2 m  s_factor=64  length=iis_element_len m  length_ad=1 m  roughness=15e-6 m  Re_lam=2000  Re_turb=4000  g=9.80665 m/s^2  wall_type=2  pr_r_coef=iis_pres_dia_value m/Pa  time_const=0.01 s  k_sh=1.4  p0=patient_pressure Pa
      settings: SourceProductBaseCode=SH  InternalSimscapePortConfiguration="{\"Bottom\":[],\"Left\":[{\"id\":\"el_A\",\"label\":\"el_A\",\"type\":\"input\"},{\"id\":\"A\",\"label\":\"A\",\"type\":\"foundation.hydraulic.hydraulic\"}],\"Right\":[{\"id\":\"el_B\",\"label\":\"el_B\",\"type\":\"input\"},{\"id\":\"B\",\"label\":\"B\",\"type\":\"foundation.hydraulic.hydraulic\"}],\"Top\":[]}"
  Pressure Sensor4 : fl_lib/Hydraulic/Hydraulic Sensors/Hydraulic Pressure Sensor
  Simulink-PS Converter : nesl_utility/Simulink-PS Converter  PhysicalDomain=network_engine_domain  SubClassName=ps_input  LeftPortType=input  RightPortType=output  PseudoPeriodic=off  Frequencies=[]  NoiseDistribution=none  NoiseParameters=[]  Unit=1  AffineConversion=off  FilteringAndDerivatives=provide  SimscapeFilterOrder=1  InputFilterTimeConstant=0.001  UdotUserProvided=0
  Simulink-PS Converter1 : nesl_utility/Simulink-PS Converter  PhysicalDomain=network_engine_domain  SubClassName=ps_input  LeftPortType=input  RightPortType=output  PseudoPeriodic=off  Frequencies=[]  NoiseDistribution=none  NoiseParameters=[]  Unit=1  AffineConversion=off  FilteringAndDerivatives=provide  SimscapeFilterOrder=1  InputFilterTimeConstant=0.001  UdotUserProvided=0
  p5 : nesl_utility/PS-Simulink Converter  PhysicalDomain=network_engine_domain  SubClassName=ps_output  LeftPortType=input  RightPortType=output  PseudoPeriodic=off  Frequencies=[]  Unit=inherit  AffineConversion=off
  p6 : nesl_utility/PS-Simulink Converter  PhysicalDomain=network_engine_domain  SubClassName=ps_output  LeftPortType=input  RightPortType=output  PseudoPeriodic=off  Frequencies=[]  Unit=inherit  AffineConversion=off
  Inlet : PMIOPort  Side=Left
  Outlet : PMIOPort  Port=2  Side=Right
  Pressure : Outport
  Flow : Outport  Port=2
  wires:
  p6/1 -> Flow/1
  p5/1 -> Pressure/1
  Elev_A/1 -> Simulink-PS Converter/1
  Elev_B/1 -> Simulink-PS Converter1/1
  connections:
  Pressure Sensor4/LConn1 -- Inlet/RConn1 -- Hydraulic Flow Rate Sensor2/LConn1
  p6/LConn1 -- Hydraulic Flow Rate Sensor2/RConn1
  Atmospheric pressure1/LConn1 -- Pressure Sensor4/RConn1
  Pressure Sensor4/RConn2 -- p5/LConn1
  Hydraulic Pipe LP with Variable Elevation/RConn2 -- Outlet/RConn1
  Hydraulic Flow Rate Sensor2/RConn2 -- Hydraulic Pipe LP with Variable Elevation/LConn2
  Simulink-PS Converter/RConn1 -- Hydraulic Pipe LP with Variable Elevation/LConn1
  Simulink-PS Converter1/RConn1 -- Hydraulic Pipe LP with Variable Elevation/RConn1

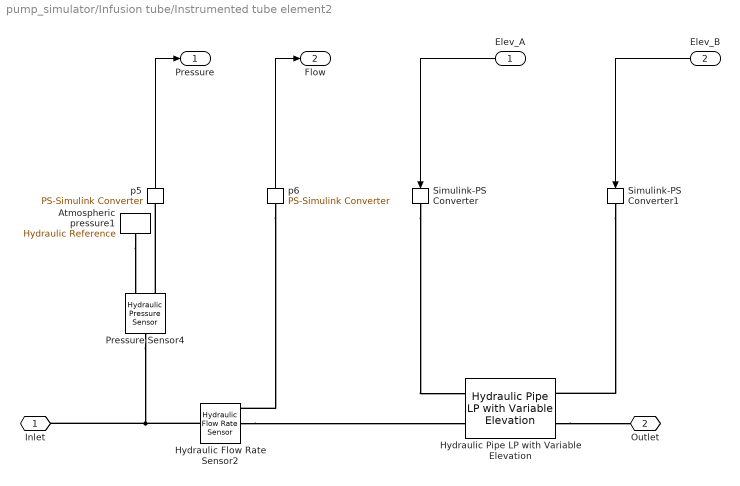
== system pump_simulator/Infusion tube/Instrumented tube element2 ==
  Elev_A : Inport
  Elev_B : Inport  Port=2
  Atmospheric pressure1 : fl_lib/Hydraulic/Hydraulic Elements/Hydraulic Reference
  Hydraulic Flow Rate Sensor2 : fl_lib/Hydraulic/Hydraulic Sensors/Hydraulic Flow Rate Sensor
  Hydraulic Pipe LP with Variable Elevation : sh_lib/Low-Pressure Blocks/Hydraulic Pipe LP with Variable Elevation  cs_type=1  d_in=iis_diameter mm  area=1e-4 m^2  D_h=1.12e-2 m  s_factor=64  length=iis_element_len m  length_ad=1 m  roughness=15e-6 m  Re_lam=2000  Re_turb=4000  g=9.80665 m/s^2  wall_type=2  pr_r_coef=iis_pres_dia_value m/Pa  time_const=0.01 s  k_sh=1.4  p0=patient_pressure Pa
      settings: SourceProductBaseCode=SH  InternalSimscapePortConfiguration="{\"Bottom\":[],\"Left\":[{\"id\":\"el_A\",\"label\":\"el_A\",\"type\":\"input\"},{\"id\":\"A\",\"label\":\"A\",\"type\":\"foundation.hydraulic.hydraulic\"}],\"Right\":[{\"id\":\"el_B\",\"label\":\"el_B\",\"type\":\"input\"},{\"id\":\"B\",\"label\":\"B\",\"type\":\"foundation.hydraulic.hydraulic\"}],\"Top\":[]}"
  Pressure Sensor4 : fl_lib/Hydraulic/Hydraulic Sensors/Hydraulic Pressure Sensor
  Simulink-PS Converter : nesl_utility/Simulink-PS Converter  PhysicalDomain=network_engine_domain  SubClassName=ps_input  LeftPortType=input  RightPortType=output  PseudoPeriodic=off  Frequencies=[]  NoiseDistribution=none  NoiseParameters=[]  Unit=1  AffineConversion=off  FilteringAndDerivatives=provide  SimscapeFilterOrder=1  InputFilterTimeConstant=0.001  UdotUserProvided=0
  Simulink-PS Converter1 : nesl_utility/Simulink-PS Converter  PhysicalDomain=network_engine_domain  SubClassName=ps_input  LeftPortType=input  RightPortType=output  PseudoPeriodic=off  Frequencies=[]  NoiseDistribution=none  NoiseParameters=[]  Unit=1  AffineConversion=off  FilteringAndDerivatives=provide  SimscapeFilterOrder=1  InputFilterTimeConstant=0.001  UdotUserProvided=0
  p5 : nesl_utility/PS-Simulink Converter  PhysicalDomain=network_engine_domain  SubClassName=ps_output  LeftPortType=input  RightPortType=output  PseudoPeriodic=off  Frequencies=[]  Unit=inherit  AffineConversion=off
  p6 : nesl_utility/PS-Simulink Converter  PhysicalDomain=network_engine_domain  SubClassName=ps_output  LeftPortType=input  RightPortType=output  PseudoPeriodic=off  Frequencies=[]  Unit=inherit  AffineConversion=off
  Inlet : PMIOPort  Side=Left
  Outlet : PMIOPort  Port=2  Side=Right
  Pressure : Outport
  Flow : Outport  Port=2
  wires:
  p6/1 -> Flow/1
  p5/1 -> Pressure/1
  Elev_A/1 -> Simulink-PS Converter/1
  Elev_B/1 -> Simulink-PS Converter1/1
  connections:
  Pressure Sensor4/LConn1 -- Inlet/RConn1 -- Hydraulic Flow Rate Sensor2/LConn1
  p6/LConn1 -- Hydraulic Flow Rate Sensor2/RConn1
  Atmospheric pressure1/LConn1 -- Pressure Sensor4/RConn1
  Pressure Sensor4/RConn2 -- p5/LConn1
  Hydraulic Pipe LP with Variable Elevation/RConn2 -- Outlet/RConn1
  Hydraulic Flow Rate Sensor2/RConn2 -- Hydraulic Pipe LP with Variable Elevation/LConn2
  Simulink-PS Converter/RConn1 -- Hydraulic Pipe LP with Variable Elevation/LConn1
  Simulink-PS Converter1/RConn1 -- Hydraulic Pipe LP with Variable Elevation/RConn1

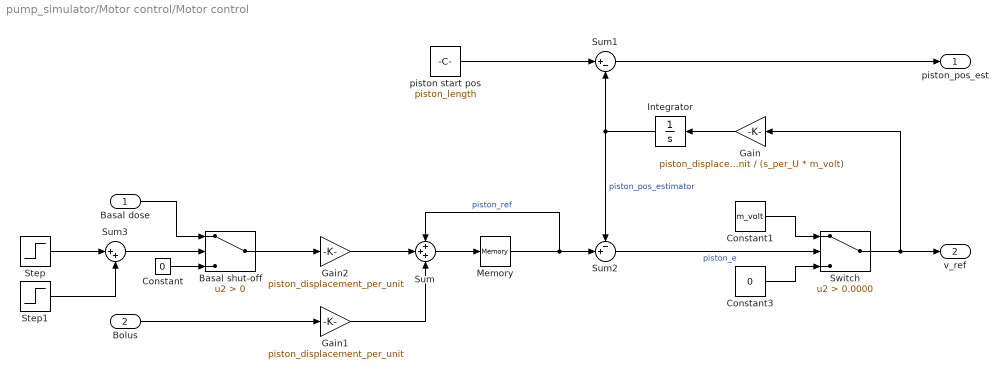
== system pump_simulator/Motor control/Motor control ==
  Basal dose : Inport
  Bolus : Inport  Port=2
  Basal shut-off : Switch  Criteria=u2 > Threshold
  Constant : Constant  Value=0
  Constant1 : Constant  Value=m_volt
  Constant3 : Constant  Value=0
  Gain : Gain  Gain=piston_displacement_per_unit / (s_per_U * m_volt)
  Gain1 : Gain  Gain=piston_displacement_per_unit
  Gain2 : Gain  Gain=piston_displacement_per_unit
  Integrator : Integrator
  Memory : Memory
  Step : Step  Time=pump_stop_time  Before=1  After=0  SampleTime=0
  Step1 : Step  Time=pump_stop_time+3600  SampleTime=0
  Sum : Sum  Inputs=+++
  Sum1 : Sum  Inputs=|+-
  Sum2 : Sum  Inputs=-+|
  Sum3 : Sum  Inputs=|++
  Switch : Switch  Criteria=u2 > Threshold  Threshold=0.0000
  piston start pos : Constant  Value=piston_length
  piston_pos_est : Outport
  v_ref : Outport  Port=2
  wires:
  Memory/1 -> Sum2/2, Sum/1  "piston_ref"
  Sum2/1 -> Switch/2  "piston_e"
  Constant3/1 -> Switch/3
  Sum/1 -> Memory/1
  Gain1/1 -> Sum/3
  Bolus/1 -> Gain1/1
  Gain2/1 -> Sum/2
  Constant1/1 -> Switch/1
  Switch/1 -> v_ref/1, Gain/1
  Gain/1 -> Integrator/1
  Integrator/1 -> Sum2/1, Sum1/2  "piston_pos_estimator"
  piston start pos/1 -> Sum1/1
  Sum1/1 -> piston_pos_est/1
  Constant/1 -> Basal shut-off/3
  Basal dose/1 -> Basal shut-off/1
  Basal shut-off/1 -> Gain2/1
  Step/1 -> Sum3/1
  Sum3/1 -> Basal shut-off/2
  Step1/1 -> Sum3/2
